simulink model "AMR_ManualModeControlUnit_23b"  (R2024a)
settings: Solver=FixedStepAuto  StartTime=0.0  StopTime=inf  RelTol=1e-3
model workspace (MAT data in the model file):
  boost_speed_multiplier = 4
  max_speed_multiplier = 7
  min_motor_rpm = 30
  vehicle_track = 877
  vehicle_wheelbase = 2367
libraries: simulink_extras x1
settings Model: Creator=matlab.cut  LastModifiedBy=matlab.cut
settings SolverCC: ConcurrentTasks=on  PositivePriorityOrder=on
settings OptimizationCC: BlockReduction=off  DefaultParameterBehavior=Inlined  OptimizeBlockIOStorage=off
settings DebuggingCC: TasksWithSamePriorityMsg=none
settings HardwareCC: ProdBitPerLong=64  ProdLongLongMode=on  ProdHWDeviceType=Intel->x86-64 (Linux 64)
settings SFSimCC: MATLABDynamicMemAlloc=off
settings RTWCC: Description=Speedgoat Real-Time Target Machine  SystemTargetFile=speedgoat.tlc  TemplateMakefile=slrealtime_default_tmf  Toolchain=Simulink Real-Time Toolchain  BuildConfiguration=Faster Runs  CodeExecutionProfiling=on  TargetLang=C++  GPUComputeCapability=3.5
settings CodeAppCC: MaxIdLength=127
settings SimulinkRealTimeTargetCC: InstructionSetFMA=off  LogToMDFFile=off

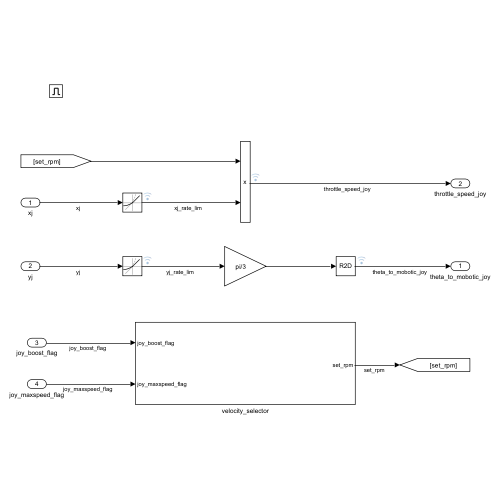
[thumbnail: Simulink's stored preview of the top-level diagram]
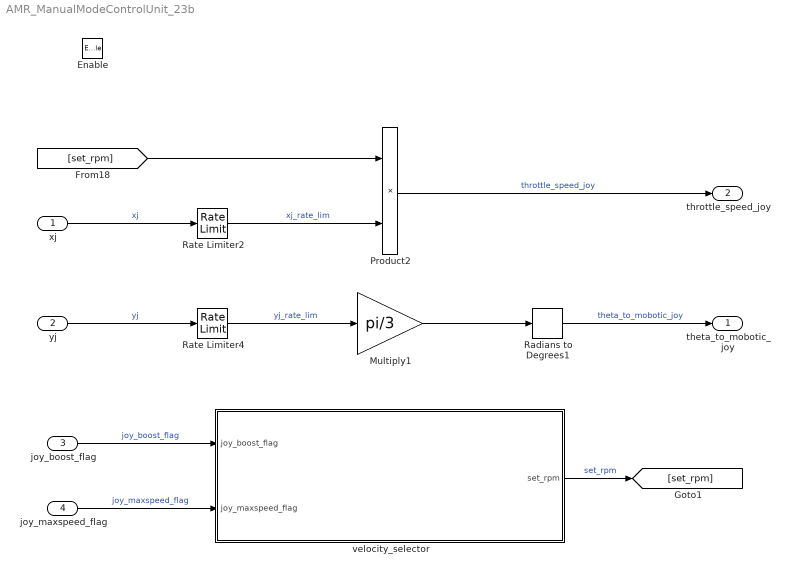
== system AMR_ManualModeControlUnit_23b ==
  xj : Inport
  yj : Inport  Port=2
  joy_boost_flag : Inport  Port=3
  joy_maxspeed_flag : Inport  Port=4
  Enable : EnablePort  OutDataTypeStr=boolean
  Multiply1 : Gain  Gain=pi/3
  Product2 : Product
  Radians to Degrees1 : simulink_extras/Transformations/Radians to Degrees
  Rate Limiter2 : RateLimiter  SampleTimeMode=inherited
  Rate Limiter4 : RateLimiter  RisingSlewLimit=0.5  FallingSlewLimit=-0.5  SampleTimeMode=inherited
  velocity_selector : Subsystem
  theta_to_mobotic_joy : Outport  OutputWhenDisabled=reset  InitialOutput=[0]
  throttle_speed_joy : Outport  Port=2  OutputWhenDisabled=reset  InitialOutput=[0]
  wires:
  yj/1 -> Rate Limiter4/1  "yj"
  Rate Limiter2/1 -> Product2/2  "xj_rate_lim"
  Product2/1 -> throttle_speed_joy/1  "throttle_speed_joy"
  [set_rpm] -> Product2/1
  Rate Limiter4/1 -> Multiply1/1  "yj_rate_lim"
  xj/1 -> Rate Limiter2/1  "xj"
  Radians to Degrees1/1 -> theta_to_mobotic_joy/1  "theta_to_mobotic_joy"
  Multiply1/1 -> Radians to Degrees1/1
  velocity_selector/1(set_rpm) -> [set_rpm]  "set_rpm"
  joy_boost_flag/1 -> velocity_selector/1(joy_boost_flag)  "joy_boost_flag"
  joy_maxspeed_flag/1 -> velocity_selector/2(joy_maxspeed_flag)  "joy_maxspeed_flag"

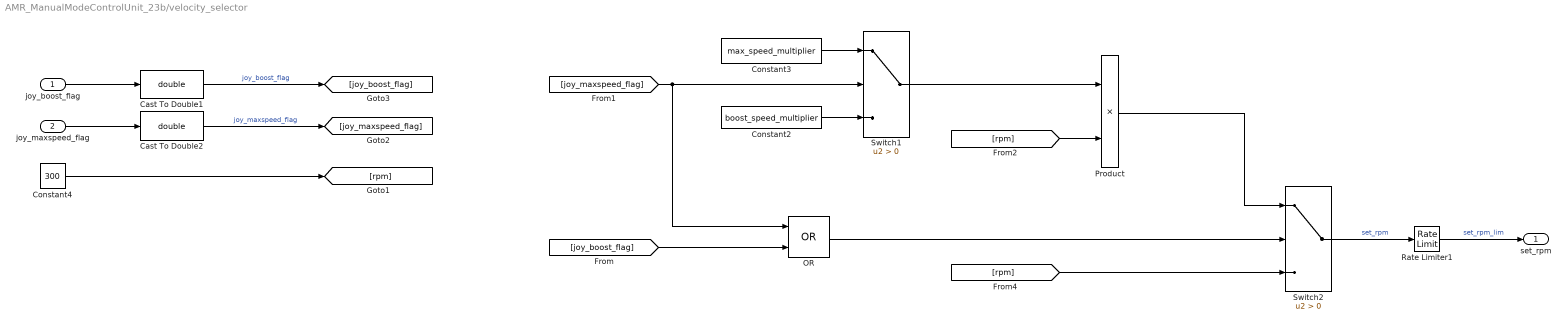
== system AMR_ManualModeControlUnit_23b/velocity_selector ==
  joy_boost_flag : Inport
  joy_maxspeed_flag : Inport  Port=2
  Cast To Double1 : DataTypeConversion  OutDataTypeStr=double  SaturateOnIntegerOverflow=off  RndMeth=Floor
  Cast To Double2 : DataTypeConversion  OutDataTypeStr=double  SaturateOnIntegerOverflow=off  RndMeth=Floor
  Constant2 : Constant  Value=boost_speed_multiplier
  Constant3 : Constant  Value=max_speed_multiplier
  Constant4 : Constant  Value=300  VectorParams1D=off
  OR : Logic  Operator=OR  AllPortsSameDT=off  OutDataTypeStr=boolean
  Product : Product
  Rate Limiter1 : RateLimiter  RisingSlewLimit=800  FallingSlewLimit=-1400  SampleTimeMode=inherited
  Switch1 : Switch  Criteria=u2 > Threshold  SaturateOnIntegerOverflow=off  InputSameDT=off
  Switch2 : Switch  Criteria=u2 > Threshold  SaturateOnIntegerOverflow=off  InputSameDT=off
  set_rpm : Outport
  wires:
  Cast To Double2/1 -> [joy_maxspeed_flag]  "joy_maxspeed_flag"
  Cast To Double1/1 -> [joy_boost_flag]  "joy_boost_flag"
  joy_boost_flag/1 -> Cast To Double1/1
  joy_maxspeed_flag/1 -> Cast To Double2/1
  [joy_boost_flag] -> OR/2
  Switch2/1 -> Rate Limiter1/1  "set_rpm"
  [joy_maxspeed_flag] -> Switch1/2, OR/1
  Constant2/1 -> Switch1/3
  [rpm] -> Product/2
  Constant4/1 -> [rpm]
  Constant3/1 -> Switch1/1
  [rpm] -> Switch2/3
  OR/1 -> Switch2/2
  Switch1/1 -> Product/1
  Product/1 -> Switch2/1
  Rate Limiter1/1 -> set_rpm/1  "set_rpm_lim"
